simulink model "test_YAN_fusion"  (R2020b)
settings: Solver=ode1  StartTime=t0  StopTime=tf  FixedStep=0.004  RelTol=1e-3  EnableMultiTasking=on
values from neighbouring files (symbols this model uses):
  IMU = IN_SENSOR.IMU1    [run_simulation.m]
undefined symbols (not defined in the file or in its folder): accel_x, accel_y, accel_z, airspeed, airspeed1, airspeed2, airspeed3, airspeed_calibrate, airspeed_indicate, airspeed_true, alt_baro, baro1, baro2, BESTPOS, delta_height, delta_lat, delta_lon, dynamic_pressure, EAS2TAS_Algo, flag, Flag, glv, gyro_x, gyro_y, gyro_z, hAcc, headAcc, height, IMU1, IMU1_Control, IMU2, IMU3, IMU4, laserDown1, laserDown2, Lat, Lon, mag1, mag2, mag_x, mag_y, mag_z, nChange, numSv, pDop, radar1, radarLongDown1, radarLongForward1, range, Range, sAcc, SNR, static_pressure, status, strength, temperature, time, ublox1, um482, vAcc ... (+3)
(part 3 of 3)

== stateflow chart test_YAN_fusion/Chart ==
  state YAN_156
    en:
    % 结构体初始化（防止编译报错）
    ins.ts = Ts;
    kf.n = 15;
    YAN.gpsvel = [0;0;0];
    en,du:
    YAN.imu = getIMU(IN_SENSOR.IMU1);
    YAN.gps = IN_SENSOR.ublox1;
    YAN.gpsvel = double([YAN.gps.velE;YAN.gps.velN;-YAN.gps.velD]);
    YAN.gpspos = double([YAN.gps.Lat*pi/180;YAN.gps.Lon*pi/180;YAN.gps.height]);
    YAN.wvm = double([YAN.imu.gyro_x,YAN.imu.gyro_y,YAN.imu.gyro_z,...
    YAN.imu.accel_x,YAN.imu.accel_y,YAN.imu.accel_z])*Ts;
    state INIT
    state RUN
      en:
      en_func;
      du:
      c_insupdate(YAN.wvm);
      c_inslever();
      c_kffk();
      c_kfupdate();
      if doMeasureUpdate
      YAN.zk = calZk();
      c_kfupdate(YAN.zk, 'M');
      c_kffeedback(1, 'avp');
      %c_kffeedback(1, 'aEDvp');
      end
    (default) -> INIT
    INIT -> RUN : after(10,sec)
  (default) -> YAN_156
  data: imu function_input; avp0 function_input; ts function_input; out function_output; imu_in function_input; davp function_output; phi function_input; dvn function_input; dpos function_input; flag function_output; eb function_input; db function_input; web function_input; wdb function_input; zk function_output; yk function_input; TimeMeasBoth function_input; varargin function_input; T_fb function_input; fbstring function_input; nts function_input; Hk function_output; pos function_input; vn function_input; IN_SENSOR input Bus: BUS_SENSOR; eulerd input; ins output Bus: BUS_NAVI_YAN_Ins; kf output Bus: BUS_NAVI_YAN_Kf; glv data_store_memory; Ts input; eth_ins local Bus: BUS_NAVI_YAN_INS_eth; YAN local Bus: BUS_NAVI_YAN_Custom size=1
  function c_insupdate(imu):
    | function c_insupdate(imu)
    | % SINS Updating Alogrithm including attitude, velocity and position
    | % updating.
    | nn = size(imu,1);
    | nts = nn*ins.ts;  nts2 = nts/2;  ins.nts = nts;
    | [phim, dvbm] = cnscl(imu,0);    % coning & sculling compensation
    | %     [phim, dvbm] = cnscl0(imu);    % coning & sculling compensation
    | phim = ins.Kg*phim-ins.eb*nts; dvbm = ins.Ka*dvbm-ins.db*nts;  % calibration
    | %% earth & angular rate updating
    | vn01 = ins.vn+ins.an*nts2; pos01 = ins.pos+ins.Mpv*vn01*nts2;  % extrapolation at t1/2
    | if ins.openloop==0, ins.eth = ethupdate(ins.eth, pos01, vn01);
    | elseif ins.openloop==1, ins.eth = ethupdate(ins.eth, ins.pos0, ins.vn0); end
    | ins.wib = phim/nts; ins.fb = dvbm/nts;  % same as trjsimu
    | ins.web = ins.wib - ins.Cnb'*ins.eth.wnie;
    | %     ins.wnb = ins.wib - ins.Cnb'*ins.eth.wnin;
    | ins.wnb = ins.wib - (ins.Cnb*rv2m(phim/2))'*ins.eth.wnin;  % 2014-11-30
    | %% (1)velocity updating
    | ins.fn = qmulv(ins.qnb, ins.fb);
    | %     ins.an = qmulv(rv2q(-ins.eth.wnin*nts2),ins.fn) + ins.eth.gcc;
    | ins.an = rotv(-ins.eth.wnin*nts2, ins.fn) + ins.eth.gcc;
    | vn1 = ins.vn + ins.an*nts;
    | %% (2)position updating
    | %     ins.Mpv = [0, 1/ins.eth.RMh, 0; 1/ins.eth.clRNh, 0, 0; 0, 0, 1];
    | ins.Mpv(4)=1/ins.eth.RMh; ins.Mpv(2)=1/ins.eth.clRNh;
    | %     ins.Mpvvn = ins.Mpv*((ins.vn+vn1)/2+(ins.an-ins.an0)*nts^2/3);  % 2014-11-30
    | ins.Mpvvn = ins.Mpv*(ins.vn+vn1)/2;
    | ins.pos = ins.pos + ins.Mpvvn*nts;
    | ins.vn = vn1;
    | ins.an0 = ins.an;
    | %% (3)attitude updating
    | ins.Cnb0 = ins.Cnb;
    | %     ins.qnb = qupdt(ins.qnb, ins.wnb*nts);  % lower accuracy than next line
    | ins.qnb = qupdt2(ins.qnb, phim, ins.eth.wnin*nts);
    | [ins.qnb, ins.att, ins.Cnb] = attsyn(ins.qnb);
    | ins.avp = [ins.att; ins.vn; ins.pos];
  function c_insinit(avp0,ts):
    | function c_insinit(avp0,ts)
    | % ins结构体初始化
    | avp0 = avp0(:);
    | [qnb0, vn0, pos0] = setvals(a2qua(avp0(1:3)), avp0(4:6), avp0(7:9));
    | ins.ts = ts; ins.nts = 1;
    | [ins.qnb, ins.vn, ins.pos] = setvals(qnb0, vn0, pos0); ins.vn0 = vn0; ins.pos0 = pos0;
    | [ins.qnb, ins.att, ins.Cnb] = attsyn(ins.qnb);  ins.Cnb0 = ins.Cnb;
    | ins.avp  = [ins.att; ins.vn; ins.pos];
    | c_ethinit(ins.pos, ins.vn);
    | ins.eth = eth_ins;
    | % 'wib,web,fn,an,Mpv,MpvCnb,Mpvvn,CW' may be very useful outside SINS,
    | % so we calucate and save them.
    | ins.wib = ins.Cnb'*ins.eth.wnin;
    | ins.fn = -ins.eth.gn;  ins.fb = ins.Cnb'*ins.fn;
    | [ins.wnb, ins.web, ins.an] = setvals(zeros(3,1));
    | ins.Mpv = [0, 1/ins.eth.RMh, 0; 1/ins.eth.clRNh, 0, 0; 0, 0, 1];
    | ins.MpvCnb = ins.Mpv*ins.Cnb;  ins.Mpvvn = ins.Mpv*ins.vn;
    | [ins.Kg, ins.Ka] = setvals(eye(3)); % calibration parameters
    | [ins.eb, ins.db] = setvals(zeros(3,1));
    | [ins.tauG, ins.tauA] = setvals(inf(3,1)); % gyro & acc correlation time
    | ins.lever = zeros(3,1); 
    | c_inslever(); % lever arm
    | ins.tDelay = 0; % time delay
    | ins.openloop = 0;
    | glv.wm_1 = zeros(3,1)';  glv.vm_1 = zeros(3,1)';  % for 'single sample+previous sample' coning algorithm
    | ins.an0 = zeros(3,1);
  function en_func:
    | function en_func()
    | YAN.avp0 = double([eulerd(2)*pi/180;eulerd(3)*pi/180;-eulerd(1)*pi/180;YAN.gpsvel;YAN.gpspos;]);
    | YAN.davp0 = c_avpseterr([30;-30;20]*1, [1;1;1]*0.3, [1;1;1]*0.1);
    | c_insinit(YAN.avp0,Ts);
    | c_imuerrset(3e2, 1e5, 3.6e0, 6e3);
    | c_kfinit(YAN.davp0,YAN.imuerr,[[1;1;2;]*0.1;[1/111e3;1/111e3;1]]);
    | % kf.Pxk(1:3,1:3) = 1e4*kf.Pxk(1:3,1:3);
    | kf.Pxk(10:15,10:15) = 1e2*kf.Pxk(10:15,10:15);
    | kf.coef_fb = 0.3 * kf.coef_fb;
    | kf.coef_fb(4:6) = 1;
  function out = getIMU(imu_in):
    | function out = getIMU(imu_in)
    | out = imu_in;
    | % from 前-右-下 to 右-前-上
    | out.accel_x = imu_in.accel_y;
    | out.accel_y = imu_in.accel_x;
    | out.accel_z = -imu_in.accel_z;
    | out.gyro_x = imu_in.gyro_y;
    | out.gyro_y = imu_in.gyro_x;
    | out.gyro_z = -imu_in.gyro_z;
  function c_inslever:
    | function c_inslever()
    | lever = ins.lever;
    | ins.CW = ins.Cnb*askew(ins.web);
    | ins.MpvCnb = ins.Mpv*ins.Cnb;
    | ins.Mpvvn = ins.Mpv*ins.vn;
    | n = size(lever,2);
    | if n>1,
    |     ins.vnL = repmat(ins.vn,1,n) + ins.CW*lever;
    |     ins.posL = repmat(ins.pos,1,n) + ins.MpvCnb*lever;
    | else  % else n==1, the following code is faster
    |     ins.vnL = ins.vn + ins.CW*lever;
    |     ins.posL = ins.pos + ins.MpvCnb*lever;
    |     ins.avpL = [ins.att; ins.vnL; ins.posL];
    | end
  function davp = c_avpseterr(phi, dvn, dpos):
    | function davp = c_avpseterr(phi, dvn, dpos)
    | davp = [phi(1:2)*glv.sec; phi(3)*glv.min; dvn; posseterr(dpos)];
  function flag = doMeasureUpdate:
    | function flag = doMeasureUpdate()
    | persistent preGpsVel
    | if isempty(preGpsVel)
    |     preGpsVel = YAN.gpsvel;
    | end
    | flag = false;
    | if any(preGpsVel ~= YAN.gpsvel)
    | %     fprintf('time: %.3f [sec] \n',t);
    |     flag = true; 
    | end
    | 
    | preGpsVel = YAN.gpsvel;
  function c_kffk:
    | function c_kffk()
    |     %% get Ft
    |     nts = ins.nts;
    | %     switch(kfmode)
    | %         case 15
    |             Ft = etm(ins);
    | %         case {18,19} % psinsdef.kffkxx, xx=18,19
    | %             Ft = etm(ins);
    | %             Ft(psinsdef.kffk, psinsdef.kffk) = 0;
    | %         case {34, 37}
    | %             Ft = etm(ins);
    | %             Ft(psinsdef.kffk,psinsdef.kffk) = 0;
    | %             Ft(1:3,20:28) = [-ins.wib(1)*ins.Cnb, -ins.wib(2)*ins.Cnb, -ins.wib(3)*ins.Cnb];
    | %             Ft(4:6,29:34) = [ins.fb(1)*ins.Cnb, ins.fb(2)*ins.Cnb(:,2:3), ins.fb(3)*ins.Cnb(:,3)];
    | %         otherwise
    | %             Ft = etm(ins);
    | % %             Ft = feval(psinsdef.typestr, psinsdef.kffktag, [{ins},varargin]);
    | %     end
    |     %% discretization
    | 	Fk = Ft*nts;
    |     if nts>0.1  % for large time interval, this may be more accurate.
    |         Fk = expm(Fk);
    |     else   % Fk = I + Ft*nts + 1/2*(Ft*nts)^2  , 2nd order expension
    |         Fk = eye(size(Ft)) + Fk;% + Fk*Fk*0.5; 
    |     end
    |     kf.Phikk_1 = Fk;
  function c_imuerrset(eb, db, web, wdb):
    | function c_imuerrset(eb, db, web, wdb)%, sqrtR0G, TauG, sqrtR0A, TauA, dKGii, dKAii, dKGij, dKAij, KA2, rxyz, dtGA)
    | % SIMU errors setting, including gyro & acc bias, noise and installation errors, etc.
    |     o31 = zeros(3,1); o33 = zeros(3);
    |     %% constant bias & random walk
    | %     if ~exist('web', 'var'), web=0; end
    | %     if ~exist('wdb', 'var'), wdb=0; end
    |     YAN.imuerr.eb(1:3) = eb*glv.dph;   YAN.imuerr.web(1:3) = web*glv.dpsh;
    |     YAN.imuerr.db(1:3) = db*glv.ug;    YAN.imuerr.wdb(1:3) = wdb*glv.ugpsHz;
    | %     %% correlated bias
    | %     if exist('sqrtR0G', 'var')
    | %         if TauG(1)==inf, YAN.imuerr.sqg(1:3) = sqrtR0G*glv.dphpsh;   % algular rate random walk !!!
    | %         elseif TauG(1)>0, YAN.imuerr.sqg(1:3) = sqrtR0G*glv.dph.*sqrt(2./TauG); YAN.imuerr.taug(1:3) = TauG; % Markov process
    | %         end
    | %     end
    | %     if exist('sqrtR0A', 'var')
    | %         if TauA(1)==inf, YAN.imuerr.sqa(1:3) = sqrtR0A*glv.ugpsh;   % specific force random walk !!!
    | %         elseif TauA(1)>0, YAN.imuerr.sqa(1:3) = sqrtR0A*glv.ug.*sqrt(2./TauA); YAN.imuerr.taua(1:3) = TauA; % Markov process
    | %         end
    | %     end
    | %     %% scale factor error
    | %     if exist('dKGii', 'var')
    | %         YAN.imuerr.dKg = setdiag(YAN.imuerr.dKg, dKGii*glv.ppm);
    | %     end
    | %     if exist('dKAii', 'var')
    | %         YAN.imuerr.dKa = setdiag(YAN.imuerr.dKa, dKAii*glv.ppm);
    | %     end
    | %     %% installation angle error
    | %     if exist('dKGij', 'var')
    | %         dKGij = ones(6,1).*dKGij*glv.sec;
    | %         YAN.imuerr.dKg(2,1) = dKGij(1); YAN.imuerr.dKg(3,1) = dKGij(2); YAN.imuerr.dKg(3,2) = dKGij(3); 
    | %         YAN.imuerr.dKg(1,2) = dKGij(4); YAN.imuerr.dKg(1,3) = dKGij(5); YAN.imuerr.dKg(2,3) = dKGij(6);
    | %     end
    | %     if exist('dKAij', 'var')
    | %         dKAij = ones(3,1).*dKAij*glv.sec;
    | %         YAN.imuerr.dKa(2,1) = dKAij(1); YAN.imuerr.dKa(3,1) = dKAij(2); YAN.imuerr.dKa(3,2) = dKAij(3); 
    | %     end
    | %     YAN.imuerr.dKga = [YAN.imuerr.dKg(:,1); YAN.imuerr.dKg(:,2);   YAN.imuerr.dKg(:,3);
    | %                    YAN.imuerr.dKa(:,1); YAN.imuerr.dKa(2:3,2); YAN.imuerr.dKa(3,3)];
    | %     %% acc 2nd scale factor error
    | %     if exist('KA2', 'var')
    | %         YAN.imuerr.KA2(1:3) = KA2*glv.ugpg2; 
    | %     end
    | %     %% acc inner-lever-arm error
    | %     if exist('rxyz', 'var')
    | %         if length(rxyz)==1, rxyz(1:6)=rxyz; end
    | %         if length(rxyz)==6, rxyz(7:9)=[0;0;0]; end 
    | %         YAN.imuerr.rx = rxyz(1:3)/100; YAN.imuerr.ry = rxyz(4:6)/100; YAN.imuerr.rz = rxyz(7:9)/100;
    | %     end
    | %     %% time-asynchrony between gyro & acc
    | %     if exist('dtGA', 'var')
    | %         YAN.imuerr.dtGA = dtGA/1000; 
    | %     end
  function zk = calZk:
    | function zk = calZk()
    | % switch kfmode
    | %     case 153
    | %         zk = [ins.pos-YAN.gpspos];
    | %     case 156
    |         zk = [ins.vn-YAN.gpsvel; ins.pos-YAN.gpspos];
    | %     case 183
    | %         dt = 0;
    | %         zk = [ins.posL-ins.Mpvvn*dt-YAN.gpspos];
    | %     case {186,196,376}
    | %         dt = 0;
    | %         zk = [ins.vnL-ins.an*dt-YAN.gpsvel; ins.posL-ins.Mpvvn*dt-YAN.gpspos];
    | %     otherwise
    | %         zk = [ins.pos-YAN.gpspos];
    | % end
    | 
    | test = 1;
  function c_kfupdate(yk, TimeMeasBoth):
    | function c_kfupdate(yk, TimeMeasBoth)
    | % Discrete-time Kalman filter.
    | %
    | % Prototype: kf = kfupdate(kf, yk, TimeMeasBoth)
    | % Inputs: kf - Kalman filter structure array
    | %         yk - measurement vector
    | %         TimeMeasBoth - described as follows,
    | %            TimeMeasBoth='T' (or nargin==1) for time updating only,
    | %            TimeMeasBoth='M' for measurement updating only,
    | %            TimeMeasBoth='B' (or nargin==2) for both time and
    | %                             measurement updating.
    | % Output: kf - Kalman filter structure array after time/meas updating
    | % Notes: (1) the Kalman filter stochastic models is
    | %      xk = Phikk_1*xk_1 + wk_1
    | %      yk = Hk*xk + vk
    | %    where E[wk]=0, E[vk]=0, E[wk*wk']=Qk, E[vk*vk']=Rk, E[wk*vk']=0
    | %    (2) If kf.adaptive=1, then use Sage-Husa adaptive method (but only for
    | %    measurement noise 'Rk'). The 'Rk' adaptive formula is:
    | %      Rk = b*Rk_1 + (1-b)*(rk*rk'-Hk*Pxkk_1*Hk')
    | %    where minimum constrain 'Rmin' and maximum constrain 'Rmax' are
    | %    considered to avoid divergence.
    | %    (3) If kf.fading>1, then use fading memory filtering method.
    | %    (4) Using Pmax&Pmin to constrain Pxk, such that Pmin<=diag(Pxk)<=Pmax.
    | %
    | % See also  kfinit, kfupdatesq, kffk, kfhk, kfc2d, kffeedback, kfplot, RLS, ekf, ukf.
    | 
    | % Copyright(c) 2009-2015, by Gongmin Yan, All rights reserved.
    | % Northwestern Polytechnical University, Xi An, P.R.China
    | % 08/12/2012, 29/08/2013, 16/04/2015, 01/06/2017, 11/03/2018
    | if nargin==0
    |     TimeMeasBoth = 'T';
    | elseif nargin==1
    |     TimeMeasBoth = 'B';
    | end
    | 
    | if TimeMeasBoth=='T'            % Time Updating
    |     kf.xk = kf.Phikk_1*kf.xk;
    |     kf.Pxk = kf.Phikk_1*kf.Pxk*kf.Phikk_1' + kf.Gammak*kf.Qk*kf.Gammak';
    | else
    |     if TimeMeasBoth=='M'        % Meas Updating
    |         kf.xkk_1 = kf.xk;
    |         kf.Pxkk_1 = kf.Pxk;
    |     elseif TimeMeasBoth=='B'    % Time & Meas Updating
    |         kf.xkk_1 = kf.Phikk_1*kf.xk;
    |         kf.Pxkk_1 = kf.Phikk_1*kf.Pxk*kf.Phikk_1' + kf.Gammak*kf.Qk*kf.Gammak';
    |     else
    |         error('TimeMeasBoth input error!');
    |     end
    |     kf.Pxykk_1 = kf.Pxkk_1*kf.Hk';
    |     kf.Py0 = kf.Hk*kf.Pxykk_1;
    |     kf.ykk_1 = kf.Hk*kf.xkk_1;
    |     kf.rk = yk-kf.ykk_1;
    |     if kf.adaptive==1  % for adaptive KF, make sure Rk is diag 24/04/2015
    |         for k=1:kf.m
    |             if yk(k)>1e10, continue; end  % 16/12/2019
    |             ry = kf.rk(k)^2-kf.Py0(k,k);
    |             if ry<kf.Rmin(k,k), ry = kf.Rmin(k,k); end
    |             if ry>kf.Rmax(k,k),     kf.Rk(k,k) = kf.Rmax(k,k);
    |             else                	kf.Rk(k,k) = (1-kf.beta)*kf.Rk(k,k) + kf.beta*ry;
    |             end
    |         end
    |         kf.beta = kf.beta/(kf.beta+kf.b);
    |     end
    |     kf.Pykk_1 = kf.Py0 + kf.Rk;
    |     kf.Kk = kf.Pxykk_1*invbc(kf.Pykk_1); % kf.Kk = kf.Pxykk_1*kf.Pykk_1^-1;
    |     kf.xk = kf.xkk_1 + kf.Kk*kf.rk;
    |     kf.Pxk = kf.Pxkk_1 - kf.Kk*kf.Pykk_1*kf.Kk';
    |     kf.Pxk = (kf.Pxk+kf.Pxk')*(kf.fading/2); % symmetrization & forgetting factor 'fading'
    |     %         if kf.adaptive==1
    |     %             krrk = kf.Kk*kf.rk*kf.rk'*kf.Kk';
    |     %             for k=3:3
    |     %                 krrki = krrk(k,k) + kf.Pxk(k,k) - kf.Pxkk_1(k,k);
    |     %                 if krrki>kf.Qmax(k,k),     kf.Qk(k,k) = kf.Qmax(k,k);
    |     %                 elseif krrki<kf.Qmin(k,k), kf.Qk(k,k) = (1-kf.beta)*kf.Qk(k,k) + kf.beta*kf.Qmin(k,k);
    |     %                 else                	kf.Qk(k,k) = (1-kf.beta)*kf.Qk(k,k) + kf.beta*krrki;
    |     %                 end
    |     %             end
    |     %         end
    | end
  function c_kfinit(varargin):
    | function c_kfinit(varargin)
    | % Kalman filter initializes for structure array 'kf', this precedure 
    | % usually includs the setting of structure fields: Qk, Rk, Pxk, Hk.
    | %
    | % Prototype: kf = kfinit(ins, varargin)
    | % Inputs: ins - SINS structure array, if not struct then nts=ins;
    | %         varargin - if any other parameters
    | % Output: kf - Kalman filter structure array
    | %
    | % See also  kfinit0, kffk, kfkk, kfupdate, kffeedback, kftypedef.
    | 
    | % Copyright(c) 2009-2014, by Gongmin Yan, All rights reserved.
    | % Northwestern Polytechnical University, Xi An, P.R.China
    | % 09/10/2013
    | [Re,deg,dph,ug,mg] = ... % just for short
    |     setvals(glv.Re,glv.deg,glv.dph,glv.ug,glv.mg); 
    | o33 = zeros(3); I33 = eye(3); 
    | % kf = [];
    | nts = ins.nts;
    | % switch(psinsdef.kfinit)
    | %     case psinsdef.kfinit153,
    | %         psinsdef.kffk = 15;  psinsdef.kfhk = 153;  psinsdef.kfplot = 15;
    | %         [davp, imuerr, rk] = setvals(varargin);
    | %         kf.Qt = diag([imuerr.web; imuerr.wdb; zeros(9,1)])^2;
    | %         kf.Rk = diag(rk)^2;
    | %         kf.Pxk = diag([davp; imuerr.eb; imuerr.db]*1.0)^2;
    | %         kf.Hk = kfhk(0);
    | %     case psinsdef.kfinit156,
    | %         psinsdef.kffk = 15;  psinsdef.kfhk = 156;  psinsdef.kfplot = 15;
    |         [davp, imuerr, rk] = setvals(varargin);
    |         kf.Qt = diag([imuerr.web; imuerr.wdb; zeros(9,1)])^2;
    |         kf.Rk = diag(rk)^2;
    |         kf.Pxk = diag([davp; imuerr.eb; imuerr.db]*1.0)^2;
    |         kf.Hk = c_kfhk();
    | %     case psinsdef.kfinit183,
    | %         psinsdef.kffk = 18;  psinsdef.kfhk = 183;  psinsdef.kfplot = 18;
    | %         [davp, imuerr, lever, r0] = setvals(varargin);
    | %         kf.Qt = diag([imuerr.web; imuerr.wdb; zeros(9+3,1)])^2;
    | %         kf.Rk = diag(r0)^2;
    | %         kf.Pxk = diag([davp; imuerr.eb; imuerr.db; lever]*1.0)^2;
    | %         kf.Hk = zeros(3,18);
    | %     case psinsdef.kfinit186,
    | %         psinsdef.kffk = 18;  psinsdef.kfhk = 186;  psinsdef.kfplot = 18;
    | %         [davp, imuerr, lever, r0] = setvals(varargin);
    | %         kf.Qt = diag([imuerr.web; imuerr.wdb; zeros(3,1); imuerr.sqg; imuerr.sqa; zeros(3,1)])^2;
    | %         kf.Rk = diag(r0)^2;
    | %         kf.Pxk = diag([davp; imuerr.eb; imuerr.db; lever]*1.0)^2;
    | %         kf.Hk = zeros(6,18);
    | %     case psinsdef.kfinit193
    | %         psinsdef.kffk = 19;  psinsdef.kfhk = 193;  psinsdef.kfplot = 19;
    | %         [davp, imuerr, lever, dT, r0] = setvals(varargin);
    | %         kf.Qt = diag([imuerr.web; imuerr.wdb; [1/Re;1/Re;1]*glv.mpsh; ...
    | %             [1;1;1]*0*glv.dphpsh; [1;1;1]*0*glv.ugpsh; [1;1;1]*0.*glv.mpsh; 0])^2;
    | %         kf.Rk = diag(r0)^2;
    | %         kf.Pxk = diag([davp; imuerr.eb; imuerr.db; lever; dT]*1.0)^2;
    | %         kf.Hk = zeros(3,19);
    | %     case psinsdef.kfinit196
    | %         psinsdef.kffk = 19;  psinsdef.kfhk = 196;  psinsdef.kfplot = 19;
    | %         [davp, imuerr, lever, dT, r0] = setvals(varargin);
    | %         kf.Qt = diag([imuerr.web; imuerr.wdb; [1/Re;1/Re;1]*glv.mpsh; ...
    | %             [1;1;1]*0*glv.dphpsh; [1;1;1]*0*glv.ugpsh; [1;1;1]*0*glv.mpsh; 0])^2;
    | %         kf.Rk = diag(r0)^2;
    | %         kf.Pxk = diag([davp; imuerr.eb; imuerr.db; lever; dT]*1.0)^2;
    | %         kf.Hk = zeros(6,19);
    | %     case psinsdef.kfinit346,
    | %         psinsdef.kffk = 34;  psinsdef.kfhk = 346;  psinsdef.kfplot = 34;
    | %         [davp, imuerr, lever, dT, r0] = setvals(varargin);
    | %         kf.Qt = diag([imuerr.web; imuerr.wdb; zeros(9+3+1+15,1)])^2;
    | %         kf.Rk = diag(r0)^2;
    | %         kf.Pxk = diag([davp; imuerr.eb; imuerr.db; lever; dT; imuerr.dKga])^2;
    | %         kf.Hk = kfhk(ins);
    | %         kf.xtau(1:psinsdef.kffk,1) = 0;
    | %     case psinsdef.kfinit376,
    | %         psinsdef.kffk = 37;  psinsdef.kfhk = 376;  psinsdef.kfplot = 37;
    | %         [davp, imuerr, lever, dT, r0] = setvals(varargin);
    | %         kf.Qt = diag([imuerr.web; imuerr.wdb; zeros(9+3+1+15+3,1)])^2;
    | %         kf.Rk = diag(r0)^2;
    | %         kf.Pxk = diag([davp; imuerr.eb; imuerr.db; lever; dT; imuerr.dKga; davp(4:6)]*10)^2;
    | %         kf.Hk = kfhk(ins);
    | %         kf.xtau(1:psinsdef.kffk,1) = 0;
    | %     otherwise,
    | %         kf = feval(psinsdef.typestr, psinsdef.kfinittag, [{ins},varargin]);
    | % end
    | c_kfinit0(nts);
  function c_kffeedback(T_fb, fbstring):
    | function c_kffeedback(T_fb, fbstring)
    | % Kalman filter state estimation feedback to SINS.
    | if kf.T_fb~=T_fb
    |     kf.T_fb = T_fb;
    |     %         kf.coef_fb = (1.0-exp(-kf.T_fb./kf.xtau));
    |     %         kf.coef_fb = ar1coefs(kf.T_fb, kf.xtau);
    |     xtau = kf.xtau;
    |     xtau(kf.xtau<kf.T_fb) = kf.T_fb;  kf.coef_fb = kf.T_fb./xtau;  %2015-2-22
    | end
    | if nargin>1 % commonly used
    |     xfb_tmp = kf.coef_fb.*kf.xk;
    |     for k=1:length(fbstring)
    |         switch fbstring(k)
    |             case 'a'
    |                 idx = 1:3; ins.qnb = qdelphi(ins.qnb, xfb_tmp(idx));
    |             case 'v'
    |                 idx = 4:6; ins.vn = ins.vn - xfb_tmp(idx);
    |             case 'p'
    |                 idx = 7:9; ins.pos = ins.pos - xfb_tmp(idx);
    |             case 'e'
    |                 idx = 10:12; ins.eb = ins.eb + xfb_tmp(idx);
    |             case 'd'
    |                 idx = 13:15; ins.db = ins.db + xfb_tmp(idx);
    | %             case 'A',
    | %                 idx = 1:2; ins.qnb = qdelphi(ins.qnb, [xfb_tmp(idx);0]);
    | %             case 'V',
    | %                 idx = 6; ins.vn(3) = ins.vn(3) - xfb_tmp(idx);
    | %             case 'P',
    | %                 idx = 9; ins.pos(3) = ins.pos(3) - xfb_tmp(idx);
    | %             case 'E',
    | %                 idx = 10:11; ins.eb(1:2) = ins.eb(1:2) + xfb_tmp(idx);
    | %             case 'D',
    | %                 idx = 15; ins.db(3) = ins.db(3) + xfb_tmp(idx);
    | %             case 'L',
    | %                 idx = 16:18; ins.lever = ins.lever + xfb_tmp(idx);
    | %             case 'T',
    | %                 idx = 19; ins.tDelay = ins.tDelay + xfb_tmp(idx);
    | %             case 'G',
    | %                 idx = 20:28; dKg = xfb_tmp(idx);  dKg = [dKg(1:3),dKg(4:6),dKg(7:9)];
    | %                 ins.Kg = (eye(3)-dKg)*ins.Kg;
    | %             case 'C',
    | %                 idx = 29:34; dKa = xfb_tmp(idx);  dKa = [dKa(1:3),[0;dKa(4:5)],[0;0;dKa(6)]];
    | %                 ins.Ka = (eye(3)-dKa)*ins.Ka;
    | %             case 'H',
    | %                 idx = [6,9,15];                         ins.vn(3) = ins.vn(3) - xfb_tmp(6);
    | %                 ins.pos(3) = ins.pos(3) - xfb_tmp(9);	ins.db(3) = ins.db(3) + xfb_tmp(15);
    |             otherwise,
    |                 error('feedback string mismatch in kf_feedback');
    |         end
    |         kf.xk(idx) = kf.xk(idx) - xfb_tmp(idx);    %
    |         kf.xfb(idx) = kf.xfb(idx) + xfb_tmp(idx);  % record total feedback
    |     end
    |     [ins.qnb, ins.att, ins.Cnb] = attsyn(ins.qnb);
    |     ins.avp = [ins.att; ins.vn; ins.pos];  % 2015-2-22
    |     return;
    | end
  function c_kfinit0(nts):
    | function c_kfinit0(nts)
    | % Always called by kfinit and initialize the remaining fields of kf.
    | % See also kfinit, kfupdate, kffeedback.
    | nState = 15;
    | nMeasure = 6;
    | kf.nts = nts;
    | [kf.m, kf.n] = size(kf.Hk);
    | kf.I = eye(nState);
    | kf.Kk = zeros(nState, nMeasure);
    | kf.xk = zeros(nState, 1);
    | kf.Qk = kf.Qt*kf.nts;
    | kf.Gammak = 1; kf.l = nState;
    | kf.fading = 1;
    | kf.adaptive = 0;
    | %     if kf.adaptive==1
    | kf.b = 0.9;
    | kf.beta = 1;
    | kf.Rmin = 0.01*kf.Rk;
    | kf.Rmax = 100*kf.Rk;
    | kf.Qmin = 0.01*kf.Qk;
    | kf.Qmax = 100*kf.Qk;
    | %
    | kf.xtau = ones(size(kf.xk))*eps;
    | kf.T_fb = 1;
    | kf.xconstrain = 0;
    | kf.pconstrain = 0;
    | kf.xfb = zeros(nState, 1);
    | %     kf.coef_fb = (1.0-exp(-kf.T_fb./kf.xtau));
    | %     kf.coef_fb = ar1coefs(kf.T_fb, kf.xtau);
    | xtau = kf.xtau;
    | xtau(kf.xtau<kf.T_fb) = kf.T_fb;  kf.coef_fb = kf.T_fb./xtau;  %2015-2-22
  function Hk = c_kfhk:
    | function Hk = c_kfhk()
    | % Establish Kalman filter measurement matrix.
    | %
    | % Prototype: Hk = kfhk(ins, varargin)
    | % Inputs: ins - SINS structure array from function 'insinit'
    | %         varargin - if any other parameters
    | % Output: Hk - measurement matrix
    | %
    | % See also  kffk, kfinit, kfupdate, kfc2d, insupdate.
    | 
    | % Copyright(c) 2009-2014, by Gongmin Yan, All rights reserved.
    | % Northwestern Polytechnical University, Xi An, P.R.China
    | % 27/03/2014, 02/02/2015
    | % global psinsdef
    | %     switch(psinsdef.kfhk)
    | %         case 153,
    | %             Hk = [zeros(3,6), eye(3), zeros(3,6)];
    | %         case 183 % glv.psinsdef.kfhkxx3
    | %             Hk = [zeros(3,6), eye(3), zeros(3,6), -ins.MpvCnb];
    | %         case 193 % glv.psinsdef.kfhkxx3
    | %             Hk = [zeros(3,6), eye(3), zeros(3,6), -ins.MpvCnb, -ins.Mpvvn];
    | %         case 343 % glv.psinsdef.kfhkxx3
    | %             Hk = [zeros(3,6), eye(3), zeros(3,6), -ins.MpvCnb, -ins.Mpvvn, zeros(3,15)];
    | %         case 373
    | %             Hk = [zeros(3,6), eye(3), zeros(3,6), -ins.MpvCnb, -ins.Mpvvn, zeros(3,18)];
    | %         case 156
    |             Hk = [zeros(6,3), eye(6), zeros(6,6)];
    | %         case 186
    | %             Hk = [zeros(6,3), eye(6), zeros(6,6), [-ins.CW;-ins.MpvCnb]];
    | %         case 196
    | %             Hk = [zeros(6,3), eye(6), zeros(6,6), [-ins.CW,-ins.an;-ins.MpvCnb,-ins.Mpvvn]];
    | %         case 346
    | %             Hk = [zeros(6,3), eye(6), zeros(6,6), [-ins.CW,-ins.an;-ins.MpvCnb,-ins.Mpvvn], zeros(6,15)];
    | %         case 376
    | %             Hk = [zeros(6,3), eye(6), zeros(6,6), [-ins.CW,-ins.an;-ins.MpvCnb,-ins.Mpvvn], zeros(6,15), [-eye(3);zeros(3)]];
    | % %         case {186, 196, 346} % glv.psinsdef.kfhkxx6
    | % %             Hk = [zeros(6,3), eye(6), zeros(6,fix(psinsdef.kfhk/10)-9)];
    | % %             Hk(1:3,16:19) = [-ins.CW, -ins.an];
    | % %             Hk(4:6,16:19) = [-ins.MpvCnb, -ins.Mpvvn];
    | % %         case 376
    | % %             Hk = [zeros(6,3), eye(6), zeros(6,fix(psinsdef.kfhk/10)-9)];
    | % %             Hk(1:3,[16:19,35:37]) = [-ins.CW, -ins.an, -eye(3)];
    | % %             Hk(4:6,16:19) = [-ins.MpvCnb, -ins.Mpvvn];
    | %         otherwise,
    | %         	Hk = feval(psinsdef.typestr, psinsdef.kfhktag, [{ins},varargin]);
    | %     end
  function c_ethinit(pos, vn):
    | function c_ethinit(pos, vn)
    | eth_ins.Re = glv.Re; eth_ins.e2 = glv.e2; eth_ins.wie = glv.wie; eth_ins.g0 = glv.g0;
    | % eth_ins = ethupdate(eth_ins, pos, vn);
    | eth_ins.pos = pos;  eth_ins.vn = vn;
    | eth_ins.sl = sin(pos(1));  eth_ins.cl = cos(pos(1));  eth_ins.tl = eth_ins.sl/eth_ins.cl;
    | eth_ins.sl2 = eth_ins.sl*eth_ins.sl;  sl4 = eth_ins.sl2*eth_ins.sl2;
    | sq = 1-eth_ins.e2*eth_ins.sl2;  RN = eth_ins.Re/sqrt(sq);
    | eth_ins.RNh = RN+pos(3);  eth_ins.clRNh = eth_ins.cl*eth_ins.RNh;
    | eth_ins.RMh = RN*(1-eth_ins.e2)/sq+pos(3);
    | %     eth_ins.wnie = [0; eth_ins.wie*eth_ins.cl; eth_ins.wie*eth_ins.sl];
    | eth_ins.wnie(2) = eth_ins.wie*eth_ins.cl; eth_ins.wnie(3) = eth_ins.wie*eth_ins.sl;
    | %     eth_ins.wnen = [-vn(2)/eth_ins.RMh; vn(1)/eth_ins.RNh; vn(1)/eth_ins.RNh*eth_ins.tl];
    | eth_ins.wnen(1) = -vn(2)/eth_ins.RMh; eth_ins.wnen(2) = vn(1)/eth_ins.RNh; eth_ins.wnen(3) = eth_ins.wnen(2)*eth_ins.tl;
    | %     eth_ins.wnin = eth_ins.wnie + eth_ins.wnen;
    | eth_ins.wnin(1) = eth_ins.wnie(1) + eth_ins.wnen(1); eth_ins.wnin(2) = eth_ins.wnie(2) + eth_ins.wnen(2); eth_ins.wnin(3) = eth_ins.wnie(3) + eth_ins.wnen(3);
    | %     eth_ins.wnien = eth_ins.wnie + eth_ins.wnin;
    | eth_ins.wnien(1) = eth_ins.wnie(1) + eth_ins.wnin(1); eth_ins.wnien(2) = eth_ins.wnie(2) + eth_ins.wnin(2); eth_ins.wnien(3) = eth_ins.wnie(3) + eth_ins.wnin(3);
    | %     eth_ins.gn = [0;0;-eth_ins.g];
    | eth_ins.g = eth_ins.g0*(1+5.27094e-3*eth_ins.sl2+2.32718e-5*sl4)-3.086e-6*pos(3); % grs80
    | eth_ins.gn(3) = -eth_ins.g;
    | %     eth_ins.gcc = eth_ins.gn - cros(eth_ins.wnien,vn); %
    | %     Gravitational/Coriolis/Centripetal acceleration eth_ins.gcc =  [
    | %     eth_ins.wnien(3)*vn(2)-eth_ins.wnien(2)*vn(3);  % faster than previous line
    | %                  eth_ins.wnien(1)*vn(3)-eth_ins.wnien(3)*vn(1);
    | %                  eth_ins.wnien(2)*vn(1)-eth_ins.wnien(1)*vn(2)+eth_ins.gn(3) ];
    | eth_ins.gcc(1) = eth_ins.wnien(3)*vn(2)-eth_ins.wnien(2)*vn(3);
    | eth_ins.gcc(2) = eth_ins.wnien(1)*vn(3)-eth_ins.wnien(3)*vn(1);
    | eth_ins.gcc(3) = eth_ins.wnien(2)*vn(1)-eth_ins.wnien(1)*vn(2)+eth_ins.gn(3);
    | eth_ins.wnie = eth_ins.wnie(:);   eth_ins.wnen = eth_ins.wnen(:);
    | eth_ins.wnin = eth_ins.wnin(:);   eth_ins.wnien = eth_ins.wnien(:);
    | eth_ins.gn = eth_ins.gn(:);       eth_ins.gcc = eth_ins.gcc(:);
